simulink model "Example_IOblock_Library_UART_Read"  (Simulink 10.3)
settings: Solver=FixedStepDiscrete  StartTime=0.0  StopTime=10.0  FixedStep=0.01  RelTol=1e-3
undefined symbols (not defined in the file): CAN_ConfigMsg, IO_Blk_Lib_TTC500, IO_CAN_WriteMsg, PopupNr, WriteMsg_CAN
libraries: IOBlock_Library_TTC580 x12, simulink x1
settings Model: Creator=hokka  LastModifiedBy=knovakovic  MultithreadedSim=on
settings DataIOCC: LimitDataPoints=on
settings OptimizationCC: InitFltsAndDblsToZero=on  LifeSpan=1  EfficientTunableParamExpr=on
settings DebuggingCC: SolverPrmCheckMsg=warning  InheritedTsInSrcMsg=none
settings HardwareCC: ProdLargestAtomicInteger=Long  ProdLargestAtomicFloat=Double  ProdIntDivRoundTo=Zero  ProdEndianess=BigEndian  ProdHWDeviceType=Texas Instruments->TMS570 Cortex-R4
settings SFSimCC: MATLABDynamicMemAlloc=off
settings RTWCC: Description=Real-Time Workshop Embedded Coder (no auto configuration)  SystemTargetFile=ert.tlc  GenCodeOnly=on  TemplateMakefile=ert_TTC580.tmf
settings CodeAppCC: IgnoreCustomStorageClasses=off  CustomSymbolStrType=$N$R$M  InternalIdentifier=Classic
settings ERTTargetCC: MultiwordLength=2048  SupportAbsoluteTime=off  SupportNonFinite=off  ERTCustomFileTemplate=example_file_process.tlc  ConvertIfToSwitch=off  SuppressUnreachableDefaultCases=off
settings ConfigComp: CovSFcnEnable=off

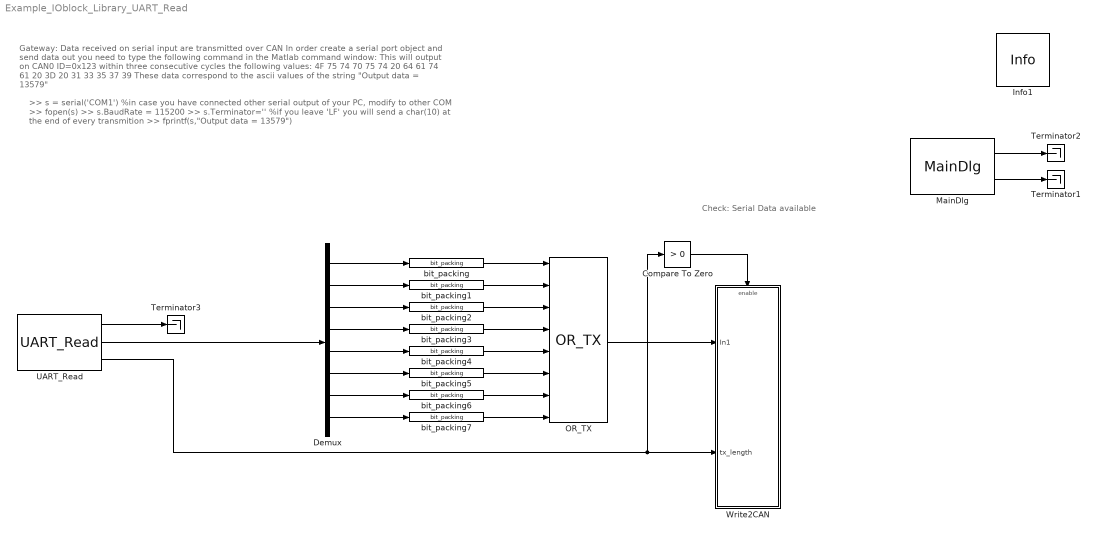
== system Example_IOblock_Library_UART_Read ==
  note: Gateway: Data received on serial input are transmitted over CAN
      | In order create a serial port object and send data out you need to type the following command in the Matlab command window:
      |
      | This will output on CAN0 ID=0x123 within three consecutive cycles the following values:
      | 4F 75 74 70 75 74 20 64
      | 61 74 61 20 3D 20 31 33
      | 35 37 39
      | These data correspond to the ascii values of the string "Output data = 13579"
  note: Check: Serial Data available
  note: >> s = serial('COM1') %in case you have connected other serial output of your PC, modify to other COM
      | >> fopen(s)
      | >> s.BaudRate = 115200
      | >> s.Terminator='' %if you leave 'LF' you will send a char(10) at the end of every transmition
      | >> fprintf(s,"Output data = 13579")
  Compare To Zero : simulink/Logic and Bit Operations/Compare To Zero  relop=>  OutDataTypeStr=boolean
  Demux : Demux  Outputs=8
  Info1 : IOBlock_Library_TTC580/Examples/Info  bla=0
      settings: SourceProductName=I/O Blocklibrary for TTC580
  MainDlg : IOBlock_Library_TTC580/System  Blocks TTC580 IOlib/MainDlg  Priority=-2147483646  SampleTime=-1  ttlib=IO_Blk_Lib_TTC500  ttDescription=MainDlg  tt_iolib_version=0.25  baudrate_CAN0=500  tseg1_CAN0=6  tseg2_CAN0=2  sjw_CAN0=1  brp_CAN0=1  baudrate_CAN1=500  tseg1_CAN1=6  tseg2_CAN1=2  sjw_CAN1=1  brp_CAN1=1  baudrate_CAN2=500  tseg1_CAN2=6  tseg2_CAN2=2  sjw_CAN2=1  brp_CAN2=1  baudrate_CAN3=500  baudrate_CAN4=500  baudrate_CAN5=500  baudrate_CAN6=500  tseg1=6  tseg2=2  sjw=1  Duration_ms=10  glitch_filter_time=180  watchdog_window_size=SAFETY_CONF_WINDOW_SIZE_100_PERCENT  watchdog_reset_behavior=SAFETY_CONF_RESETS_DISABLED  brp=0  Enable_sending_DM1_of_J1939=off  DM1_Channel=IO_CAN_CHANNEL_0  J1939SorceAddress=0  DM2_Basis_Address=63488  Show_version_information=off  Major_Number=0  Minor_Number=1  Revison_Number=1  Node_Number=1  Enable_Reset_by_TTCDownloader=on  bFlashOverEthernet=off  Enable_CCP=off  CRO_ID=hex2dec('101')  DTO_ID=hex2dec('102')  CCP_Station_Addr_raw=1  CCP_Station_ID=ECU00001  CPP_channel=IO_CAN_CHANNEL_0  CPP_id_format=IO_CAN_STD_FRAME  bEnable_DAQ0=off  bEnable_DAQ1_2=off  ODT_total=10  bEnable_ErrorCBAction=off  bDIAG_ERR_DISABLE_SSW0=off  bDIAG_ERR_DISABLE_SSW1=off  bDIAG_ERR_DISABLE_SSW2=off
      settings: SourceProductName=I/O Blocklibrary for TTC580
  OR_TX : IOBlock_Library_TTC580/CAN  Blocks TTC580 IOlib/OR_TX  logicop=OR  UseBitMask=off  NumInputPorts=8  BitMask=bin2dec('11011001')  BitMaskRealWorld=Stored Integer
      settings: SourceProductName=I/O Blocklibrary for TTC580
  Terminator1 : Terminator
  Terminator2 : Terminator
  Terminator3 : Terminator
  UART_Read : IOBlock_Library_TTC580/UART TTC580 IOlib/UART_Read  Priority=200  SampleTime=-1  ttlib=IO_Blk_Lib_TTC500  ttDescription=UART_Read  tt_iolib_version=0.25  size_of_data=8  Show_additional_information=off  baudrate=115200  dbits=8  par=IO_UART_PARITY_NONE  sbits=1
      settings: SourceProductName=I/O Blocklibrary for TTC580
  Write2CAN : Subsystem
  bit_packing : IOBlock_Library_TTC580/CAN  Blocks TTC580 IOlib/bit_packing  SampleTime=-1  ttlib=IO_Blk_Lib_TTC500  ttDescription=bit_packing  tt_iolib_version=0.26  Endianness=little  Format=unsigned  Inversion=off  Startbit=0  Width_bits=8  Factor=1.0  Offset=0.0
      settings: SourceProductName=I/O Blocklibrary for TTC580
  bit_packing1 : IOBlock_Library_TTC580/CAN  Blocks TTC580 IOlib/bit_packing  SampleTime=-1  ttlib=IO_Blk_Lib_TTC500  ttDescription=bit_packing  tt_iolib_version=0.26  Endianness=little  Format=unsigned  Inversion=off  Startbit=8  Width_bits=8  Factor=1.0  Offset=0.0
      settings: SourceProductName=I/O Blocklibrary for TTC580
  bit_packing2 : IOBlock_Library_TTC580/CAN  Blocks TTC580 IOlib/bit_packing  SampleTime=-1  ttlib=IO_Blk_Lib_TTC500  ttDescription=bit_packing  tt_iolib_version=0.26  Endianness=little  Format=unsigned  Inversion=off  Startbit=16  Width_bits=8  Factor=1.0  Offset=0.0
      settings: SourceProductName=I/O Blocklibrary for TTC580
  bit_packing3 : IOBlock_Library_TTC580/CAN  Blocks TTC580 IOlib/bit_packing  SampleTime=-1  ttlib=IO_Blk_Lib_TTC500  ttDescription=bit_packing  tt_iolib_version=0.26  Endianness=little  Format=unsigned  Inversion=off  Startbit=24  Width_bits=8  Factor=1.0  Offset=0.0
      settings: SourceProductName=I/O Blocklibrary for TTC580
  bit_packing4 : IOBlock_Library_TTC580/CAN  Blocks TTC580 IOlib/bit_packing  SampleTime=-1  ttlib=IO_Blk_Lib_TTC500  ttDescription=bit_packing  tt_iolib_version=0.26  Endianness=little  Format=unsigned  Inversion=off  Startbit=32  Width_bits=8  Factor=1.0  Offset=0.0
      settings: SourceProductName=I/O Blocklibrary for TTC580
  bit_packing5 : IOBlock_Library_TTC580/CAN  Blocks TTC580 IOlib/bit_packing  SampleTime=-1  ttlib=IO_Blk_Lib_TTC500  ttDescription=bit_packing  tt_iolib_version=0.26  Endianness=little  Format=unsigned  Inversion=off  Startbit=40  Width_bits=8  Factor=1.0  Offset=0.0
      settings: SourceProductName=I/O Blocklibrary for TTC580
  bit_packing6 : IOBlock_Library_TTC580/CAN  Blocks TTC580 IOlib/bit_packing  SampleTime=-1  ttlib=IO_Blk_Lib_TTC500  ttDescription=bit_packing  tt_iolib_version=0.26  Endianness=little  Format=unsigned  Inversion=off  Startbit=48  Width_bits=8  Factor=1.0  Offset=0.0
      settings: SourceProductName=I/O Blocklibrary for TTC580
  bit_packing7 : IOBlock_Library_TTC580/CAN  Blocks TTC580 IOlib/bit_packing  SampleTime=-1  ttlib=IO_Blk_Lib_TTC500  ttDescription=bit_packing  tt_iolib_version=0.26  Endianness=little  Format=unsigned  Inversion=off  Startbit=56  Width_bits=8  Factor=1.0  Offset=0.0
      settings: SourceProductName=I/O Blocklibrary for TTC580
  wires:
  MainDlg/1 -> Terminator2/1
  MainDlg/2 -> Terminator1/1
  UART_Read/1 -> Terminator3/1
  UART_Read/3 -> Compare To Zero/1, Write2CAN/2(tx_length)
  Demux/1 -> bit_packing/1
  Demux/2 -> bit_packing1/1
  Demux/3 -> bit_packing2/1
  Demux/4 -> bit_packing3/1
  Demux/5 -> bit_packing4/1
  Demux/6 -> bit_packing5/1
  Demux/7 -> bit_packing6/1
  Demux/8 -> bit_packing7/1
  bit_packing3/1 -> OR_TX/4
  bit_packing4/1 -> OR_TX/5
  bit_packing2/1 -> OR_TX/3
  bit_packing5/1 -> OR_TX/6
  bit_packing1/1 -> OR_TX/2
  bit_packing6/1 -> OR_TX/7
  bit_packing/1 -> OR_TX/1
  bit_packing7/1 -> OR_TX/8
  UART_Read/2 -> Demux/1
  OR_TX/1 -> Write2CAN/1(In1)
  Compare To Zero/1 -> Write2CAN/Enable

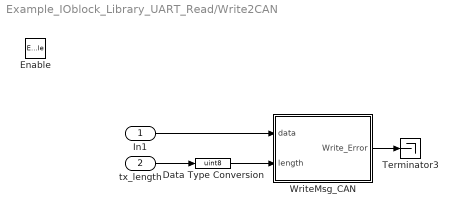
== system Example_IOblock_Library_UART_Read/Write2CAN ==
  In1 : Inport
  tx_length : Inport  Port=2
  Enable : EnablePort
  Data Type Conversion : DataTypeConversion  OutDataTypeStr=uint8
  Terminator3 : Terminator
  WriteMsg_CAN : Subsystem  LoadFcn=|  mask(WriteMsg_CAN_Code){SampleTime=-1, ttlib=IO_Blk_Lib_TTC500, ttDescription=WriteMsg_CAN, tt_iolib_version=0.26, channel=IO_CAN_CHANNEL_0, mode=IO_CAN_MSG_WRITE, id_format=IO_CAN_STD_FRAME, id=hex2dec('123'), length=8}
      | try
      | %
      | %Upgrade Information - standard BEGIN
      | new_color = 'blue';
      | new_ver = '0.26';
      | act_ver = get_param(gcb,'tt_iolib_version');
      | if not(strcmp(act_ver,new_ver))
      |     disp(['Upgrade block: ',gcb,char(10),'       Version: ',act_ver,' to ',new_ver]);
      |     %switch - case for specific upgrade information e.g. additional parameter required 
      |     %Change appearance and version information
      |     set_param(gcb,'ForegroundColor',new_color);
      |     set_param(gcb,'tt_iolib_version',new_ver);
      | end
      | %Upgrade Information - standard END
      | catch
      | %Standard catch section BEGIN
      | errordlg('An error occurred in a callback of the TTC580-BlockLib. Please open the Diagnostic Viewer for further details');
      | disp(' ');
      | disp('------------------------------------------------------------');
      | disp('An error occurred in a callback of the TTC580-BlockLib.');
      | disp(['Please check the parameters in the mask of ',gcb]);
      | disp('If you do not encounter any violations, then please '); 
      | disp('copy the following lines and report this to support@ttcontrol.com ');
      | disp('<< begin of error message dump >>');
      | disp(['Version of TTC580-BlockLib: ', get_param(gcb,'tt_iolib_version')]);
      | disp(get_param(gcb,'ttDescription'));
      | disp(gcb);
      | x=lasterror;disp(x.message);
      | disp(get_param(gcb,'MaskValues'));
      | disp(version);
      | disp(computer);
      | disp('<< end of error message dump >>');
      | disp('------------------------------------------------------------');
      | disp(' ');
      | %Standard catch section END
      | end
      mask help: Transmits a CAN message, using the given channel and message object.
      mask init:
      | try
      | %%CT>
      | TAG_loc = get_param(gcb,'Tag');
      | if ~isempty(TAG_loc),[~,y]=regexp(TAG_loc,'(^[a-zA-Z0-9_]*)');
      |     if isempty(y) || y~=builtin('length',(TAG_loc)) %don't use length() alone!
      |         error(['The Tag: ',TAG_loc,' needs to start with a letter and may only contain the characters 0-9,a-Z,_ .']);
      | end,end
      | x=find_system(gcbh,'FollowLinks','on','LookUnderMasks','on','BlockType','S-Function');
      | for i=1:builtin('length',(x)) %don't use length() alone!
      |     set_param(x(i),'Tag',TAG_loc);
      | end
      | %<CT%
      | 
      | catch
      | %Standard catch section BEGIN
      | errordlg('An error occurred in a callback of the TTC580-BlockLib. Please open the Diagnostic Viewer for further details');
      | disp(' ');
      | disp('------------------------------------------------------------');
      | disp('An error occurred in a callback of the TTC580-BlockLib.');
      | disp(['Please check the parameters in the mask of ',gcb]);
      | disp('If you do not encounter any violations, then please '); 
      | disp('copy the following lines and report this to support@ttcontrol.com ');
      | disp('<< begin of error message dump >>');
      | disp(['Version of TTC580-BlockLib: ', get_param(gcb,'tt_iolib_version')]);
      | disp(get_param(gcb,'ttDescription'));
      | disp(gcb);
      | x=lasterror;disp(x.message);
      | disp(get_param(gcb,'MaskValues'));
      | disp(version);
      | disp(computer);
      | disp('<< end of error message dump >>');
      | disp('------------------------------------------------------------');
      | disp(' ');
      | %Standard catch section END
      | end
      settings: CopyFcn=%deleted
      mask Help:
      | Help for the block parameters may be found in the description of the drivers within the system manual of the TTC5XX.
      | <br>Verification:  This block supports verification capabilities. To activate these, you need to specify a Tag in the Block Properties and use ert_TTC580_Verification.tmf for the target makefile in the Configuration Parameters. In the generated code the parameters of the driver function appear as constants with the identifiers  [Tag]__[Description]__[Parameter], which may be accessed for verification (e.g. over CCP). The name of these identifiers and their setting may be inspected in the file IOLib_ParameterValidation_[model].txt, which is generated during code generation.
      mask TypeOptions channel: IO_CAN_CHANNEL_0  | IO_CAN_CHANNEL_1 | IO_CAN_CHANNEL_2 | IO_CAN_CHANNEL_3 | IO_CAN_CHANNEL_4 | IO_CAN_CHANNEL_5 | IO_CAN_CHANNEL_6
      mask Callback channel: %
      mask Callback mode: %
      mask TypeOptions id_format: IO_CAN_STD_FRAME | IO_CAN_EXT_FRAME
      mask Callback id_format: %
      mask Callback id: %
      mask Callback length: %
  wires:
  WriteMsg_CAN/1(Write_Error) -> Terminator3/1
  In1/1 -> WriteMsg_CAN/1(data)
  tx_length/1 -> Data Type Conversion/1
  Data Type Conversion/1 -> WriteMsg_CAN/2(length)

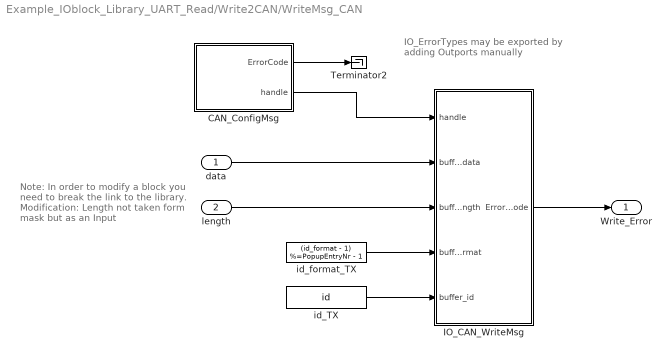
== system Example_IOblock_Library_UART_Read/Write2CAN/WriteMsg_CAN ==
  note: Note: In order to modify a block
      | you need to break the link to the
      | library.
      | Modification: Length not taken form
      | mask but as an Input
  note: IO_ErrorTypes may be exported
      | by adding Outports manually
  data : Inport
  length : Inport  Port=2
  CAN_ConfigMsg : Subsystem  LoadFcn=|  mask(CAN_ConfigMsg_Code){SampleTime=-1, ttlib=IO_Blk_Lib_TTC500, ttDescription=CAN_ConfigMsg, tt_iolib_version=0.19, channel=channel, mode=mode, id_format=(id_format-1) %PopupNr - 1, id=id, ac_mask=['0x',dec2hex((id_format==1)*hex2dec('7FF')+(id_format==2)*hex2dec('1FFFFFFF')),'U']; %id_format = PopupNr}
      | try
      | %
      | %Upgrade Information - standard BEGIN
      | new_color = 'blue';
      | new_ver = '0.19';
      | act_ver = get_param(gcb,'tt_iolib_version');
      | if not(strcmp(act_ver,new_ver))
      |     disp(['Upgrade block: ',gcb,char(10),'       Version: ',act_ver,' -> ',new_ver]);
      |     %switch - case for specific upgrade information e.g. additional parameter required 
      |     %Change appearance and version information
      |     set_param(gcb,'ForegroundColor',new_color);
      |     set_param(gcb,'tt_iolib_version',new_ver);
      | end
      | %Upgrade Information - standard END
      | catch
      | %Standard catch section BEGIN 
      | disp(' ');
      | disp('------------------------------------------------------------');
      | disp('An error occurred in a callback of the TTC580-BlockLib.');
      | disp(['Please check the parameters in the mask of ',gcb]);
      | disp('If you do not encounter any violations, then please '); 
      | disp('copy the following lines and report this to support@ttcontrol.com ');
      | disp('<< begin of error message dump >>');
      | disp(['Version of TTC580-BlockLib: ', get_param(gcb,'tt_iolib_version')]);
      | disp(get_param(gcb,'ttDescription'));
      | disp(gcb);
      | x=lasterror;disp(x.message);
      | disp(get_param(gcb,'MaskValues'));
      | disp(version);
      | disp(computer);
      | disp('<< end of error message dump >>');
      | disp('------------------------------------------------------------');
      | disp(' ');
      | %Standard catch section END
      | end
      mask help: Configures a message object for the given CAN channel.
      mask init:
      | %
      settings: CopyFcn=%deleted
      mask Help: web(which('IO_CAN.h'))
      mask Callback channel: %
      mask Callback mode: %
      mask Callback id_format: %
      mask Callback id: %
      mask Callback ac_mask: %
  IO_CAN_WriteMsg : Subsystem  LoadFcn=|  mask(IO_CAN_WriteMsg_Code){SampleTime=-1, ttlib=IO_Blk_Lib_TTC500, ttDescription=IO_CAN_WriteMsg, tt_iolib_version=0.19}
      | try
      | %
      | %Upgrade Information - standard BEGIN
      | new_color = 'blue';
      | new_ver = '0.19';
      | act_ver = get_param(gcb,'tt_iolib_version');
      | if not(strcmp(act_ver,new_ver))
      |     disp(['Upgrade block: ',gcb,char(10),'       Version: ',act_ver,' -> ',new_ver]);
      |     %switch - case for specific upgrade information e.g. additional parameter required 
      |     %Change appearance and version information
      |     set_param(gcb,'ForegroundColor',new_color);
      |     set_param(gcb,'tt_iolib_version',new_ver);
      | end
      | %Upgrade Information - standard END
      | catch
      | %Standard catch section BEGIN 
      | disp(' ');
      | disp('------------------------------------------------------------');
      | disp('An error occurred in a callback of the TTC580-BlockLib.');
      | disp(['Please check the parameters in the mask of ',gcb]);
      | disp('If you do not encounter any violations, then please '); 
      | disp('copy the following lines and report this to support@ttcontrol.com ');
      | disp('<< begin of error message dump >>');
      | disp(['Version of TTC580-BlockLib: ', get_param(gcb,'tt_iolib_version')]);
      | disp(get_param(gcb,'ttDescription'));
      | disp(gcb);
      | x=lasterror;disp(x.message);
      | disp(get_param(gcb,'MaskValues'));
      | disp(version);
      | disp(computer);
      | disp('<< end of error message dump >>');
      | disp('------------------------------------------------------------');
      | disp(' ');
      | %Standard catch section END
      | end
      mask help: Transmits a CAN message, using the given channel and message object.
      mask init:
      | %
      settings: CopyFcn=%deleted
      mask Help: web(which('IO_CAN.h'))
  Terminator2 : Terminator
  id_TX : Constant  Value=id  OutDataTypeStr=uint32
  id_format_TX : Constant  Value=(id_format - 1) %=PopupEntryNr - 1  OutDataTypeStr=Inherit: Inherit via back propagation
  Write_Error : Outport  VectorParamsAs1DForOutWhenUnconnected=off
  wires:
  id_TX/1 -> IO_CAN_WriteMsg/5(buffer_id)
  id_format_TX/1 -> IO_CAN_WriteMsg/4(buffer_id_format)
  length/1 -> IO_CAN_WriteMsg/3(buffer_length)
  data/1 -> IO_CAN_WriteMsg/2(buffer_data)
  CAN_ConfigMsg/2(handle) -> IO_CAN_WriteMsg/1(handle)
  IO_CAN_WriteMsg/1(ErrorCode) -> Write_Error/1
  CAN_ConfigMsg/1(ErrorCode) -> Terminator2/1

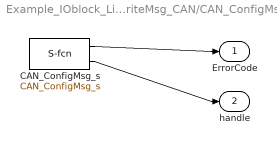
== system Example_IOblock_Library_UART_Read/Write2CAN/WriteMsg_CAN/CAN_ConfigMsg ==
  CAN_ConfigMsg_s : S-Function  FunctionName=CAN_ConfigMsg_s  Parameters=SampleTime,channel,mode,id_format,id,ac_mask  SFunctionDeploymentMode=off  EnableBusSupport=off
  ErrorCode : Outport  VectorParamsAs1DForOutWhenUnconnected=off
  handle : Outport  Port=2  VectorParamsAs1DForOutWhenUnconnected=off
  wires:
  CAN_ConfigMsg_s/1 -> ErrorCode/1
  CAN_ConfigMsg_s/2 -> handle/1

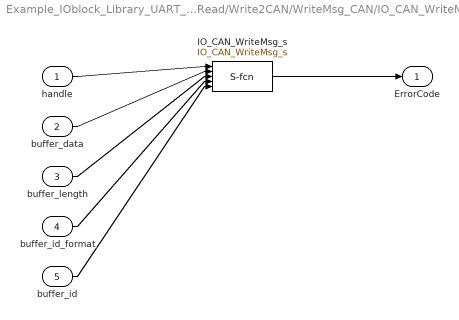
== system Example_IOblock_Library_UART_Read/Write2CAN/WriteMsg_CAN/IO_CAN_WriteMsg ==
  handle : Inport
  buffer_data : Inport  Port=2
  buffer_length : Inport  Port=3
  buffer_id_format : Inport  Port=4
  buffer_id : Inport  Port=5
  IO_CAN_WriteMsg_s : S-Function  FunctionName=IO_CAN_WriteMsg_s  Parameters=SampleTime  SFunctionDeploymentMode=off  EnableBusSupport=off
  ErrorCode : Outport  VectorParamsAs1DForOutWhenUnconnected=off
  wires:
  handle/1 -> IO_CAN_WriteMsg_s/1
  buffer_data/1 -> IO_CAN_WriteMsg_s/2
  buffer_length/1 -> IO_CAN_WriteMsg_s/3
  buffer_id_format/1 -> IO_CAN_WriteMsg_s/4
  buffer_id/1 -> IO_CAN_WriteMsg_s/5
  IO_CAN_WriteMsg_s/1 -> ErrorCode/1
